simulink model "STLA_6_30"  (R2025a)
settings: Solver=ode3  StartTime=0.0  StopTime=2474  FixedStep=0.01  RelTol=1e-3
model workspace (MAT data in the model file):
  qw = 0.5
libraries: simulink x5, svdutilitieslib x2, instrumentlib x2, autolibshared x1, pid_lib x1
settings Model: Creator=王刚  LastModifiedBy=王刚
settings SolverCC: AlgebraicLoopSolver=TrustRegion
settings RTWCC: DLArmComputeVersion=19.05

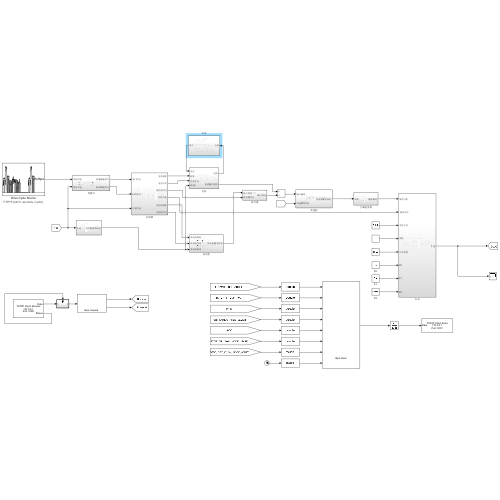
[thumbnail: Simulink's stored preview of the top-level diagram]
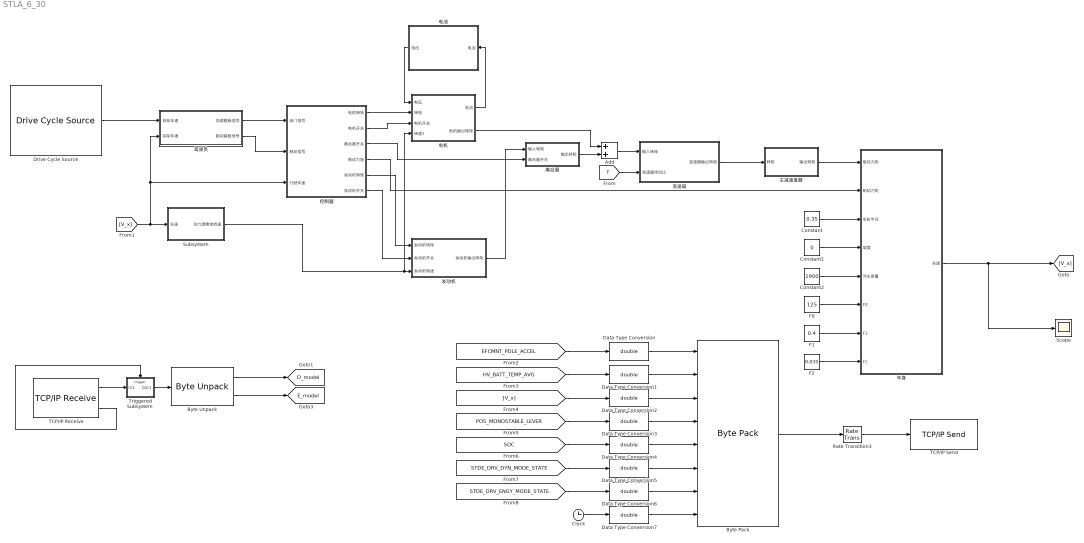
== system STLA_6_30 ==
  Add : Sum
  Byte Pack : svdutilitieslib/Byte Pack  maskPackedDataType=uint8  datatypes={'double', 'double', 'double', 'double', 'double', 'double', 'double', 'double'}  byteAlign=1  blockPlatform=tic2000
  Byte Unpack : svdutilitieslib/Byte Unpack  dimensions={[1] [1]}  datatypes={'double', 'double'}  byteAlign=1  blockPlatform=tic2000
  Clock : Clock
  Constant : Constant  Value=0.35
  Constant1 : Constant  Value=0
  Constant2 : Constant  Value=1900
  Data Type Conversion{,1..7} (8 alike) : DataTypeConversion  OutDataTypeStr=double  SaturateOnIntegerOverflow=off  RndMeth=Floor
  Drive Cycle Source : autolibshared/Drive Cycle Source  cycleVar=FTP75  fileVar=cycleFTP75.mat  tfinal="2474  seconds, Cyclic"  cycleRepeat=on  outAccPort=off  outGearPort=off  gearList=No gear data  t_wot1=5  xdot_woto=0  xdot_wot1=30  t_wot2=20  xdot_wot2=0  t_wotend=30  srcUnit=m/s  outUnit=km/h  srcAccUnit=m/s/s  outAccUnit=m/s^2  dt=0  aMode=1  faultOption=off  velBnd=2  velBndUnit=mph  inUnit=m/s  timeBnd=1  failOption=off  stopSim=off  maxFaultCnt=10  maxFaultTime=2  maxTotFaultTime=15  traceOption=off  dtTrace=1  traceWindow=10  lastDCname=FTP75  lastOutUnit=mph  lastDT=0  lastTB=1  lastSB=2  forceCalcBound=off
  F0 : Constant  Value=125
  F1 : Constant  Value=0.4
  F2 : Constant  Value=0.035
  Rate Transition3 : RateTransition  OutPortSampleTime=0.1
  Scope : Scope
      settings: ActiveDisplayYMinimum=-11.4831  ActiveDisplayYMaximum=103.3483  DataLoggingVariableName=ScopeData5  DataLoggingSaveFormat=Array
  Subsystem : Subsystem
  TCP/IP Receive : instrumentlib/TCP//IP Receive  Host=127.0.0.1  Port=5000  DataSize=16  DataType=uint8  ASCIIFormatting=%f  Terminator=LF  CustomTerminator=10  ByteOrder=big-endian  EnableBlockingMode=off  Timeout=0.01  SampleTime=0.01  SimulateUsing=Interpreted execution
  TCP/IP Send : instrumentlib/TCP//IP Send  Host=127.0.0.1  Port=5001  ByteOrder=big-endian  EnableBlockingMode=off  Timeout=10  TransferDelay=on  SimulateUsing=Interpreted execution
  Triggered Subsystem : Subsystem  TreatAsAtomicUnit=on
  主减速度器 : Subsystem
  发动机 : Subsystem
  变速箱 : Subsystem
  控制器 : Subsystem
  电机 : Subsystem
  电池 : Subsystem
  离合器 : Subsystem
  车身 : Subsystem
  驾驶员 : Subsystem
  tag scope: D_model=global, E_model=global
  wires:
  驾驶员/1(加速踏板信号) -> 控制器/1(油门信号)
  驾驶员/2(制动踏板信号) -> 控制器/2(制动信号)
  Constant/1 -> 车身/3(车轮半径)
  Constant1/1 -> 车身/4(坡度)
  Constant2/1 -> 车身/5(汽车质量)
  F0/1 -> 车身/6(F0)
  F1/1 -> 车身/7(F1)
  F2/1 -> 车身/8(F2)
  变速箱/1(变速器输出转矩) -> 主减速度器/1(转矩)
  主减速度器/1(输出转矩) -> 车身/1("驱动力矩 ")
  控制器/5(发动机转矩) -> 发动机/1(发动机转矩)
  控制器/6(发动机开关) -> 发动机/2(发动机开关)
  控制器/1(电机转矩) -> 电机/2(转矩)
  控制器/2(电机开关) -> 电机/3(电机开关)
  控制器/3(离合器开关) -> 离合器/2(离合器开关)
  控制器/4(制动力矩) -> 车身/2(" 制动力矩")
  电池/1(电压) -> 电机/1(电压)
  离合器/1(输出转矩) -> Add/2
  Add/1 -> 变速箱/1(输入转矩)
  [T] -> 变速箱/2(变速器传动比)
  车身/1(车速) -> [V_x], Scope/1
  [V_x] -> 驾驶员/2(实际车速), 控制器/3(行驶车速), Subsystem/1(车速)
  电机/1(电流) -> 电池/1(电流)
  电机/2(电机输出转矩) -> Add/1
  发动机/1(发动机输出转矩) -> 离合器/1(输入转矩)
  Subsystem/1(动力源需求转速) -> 电机/4(转速1), 发动机/3(发动机转速)
  Drive Cycle Source/1 -> 驾驶员/1(目标车速)
  Triggered Subsystem/1(Out1) -> Byte Unpack/1
  Byte Unpack/1 -> [D_model]
  Byte Unpack/2 -> [E_model]
  TCP/IP Receive/1 -> Triggered Subsystem/1(In1)
  TCP/IP Receive/2 -> Triggered Subsystem/Trigger
  [EFCMNT_PDLE_ACCEL] -> Data Type Conversion/1
  [STDE_DRV_ENGY_MODE_STATE] -> Data Type Conversion6/1
  [STDE_DRV_DYN_MODE_STATE] -> Data Type Conversion5/1
  [SOC] -> Data Type Conversion4/1
  [V_x] -> Data Type Conversion2/1
  [POS_MONOSTABLE_LEVER] -> Data Type Conversion3/1
  [HV_BATT_TEMP_AVG] -> Data Type Conversion1/1
  Byte Pack/1 -> Rate Transition3/1
  Rate Transition3/1 -> TCP/IP Send/1
  Clock/1 -> Data Type Conversion7/1
  Data Type Conversion/1 -> Byte Pack/1
  Data Type Conversion1/1 -> Byte Pack/2
  Data Type Conversion2/1 -> Byte Pack/3
  Data Type Conversion3/1 -> Byte Pack/4
  Data Type Conversion4/1 -> Byte Pack/5
  Data Type Conversion5/1 -> Byte Pack/6
  Data Type Conversion6/1 -> Byte Pack/7
  Data Type Conversion7/1 -> Byte Pack/8

== system STLA_6_30/Subsystem ==
  车速 : Inport
  " " : Constant  Value=0.377
  Product : Product  Inputs=***//
  主减速器传动比 : Constant  Value=4.88
  车轮半径 : Constant  Value=0.25
  动力源需求转速 : Outport
  tag scope: rmp=global
  wires:
  Product/1 -> [rmp], 动力源需求转速/1
  车速/1 -> Product/1
  " "/1 -> Product/5
  主减速器传动比/1 -> Product/2
  车轮半径/1 -> Product/4
  [T] -> Product/3

== system STLA_6_30/Triggered Subsystem ==
  In1 : Inport
  Trigger : TriggerPort  VariantControl=(inherit)
  Out1 : Outport
  wires:
  In1/1 -> Out1/1

== system STLA_6_30/主减速度器 ==
  转矩 : Inport
  Product : Product
  主减速器传动比 : Constant  Value=4.88
  传动效率 : Gain  Gain=0.9
  输出转矩 : Outport
  wires:
  转矩/1 -> Product/1
  主减速器传动比/1 -> Product/2
  Product/1 -> 传动效率/1
  传动效率/1 -> 输出转矩/1

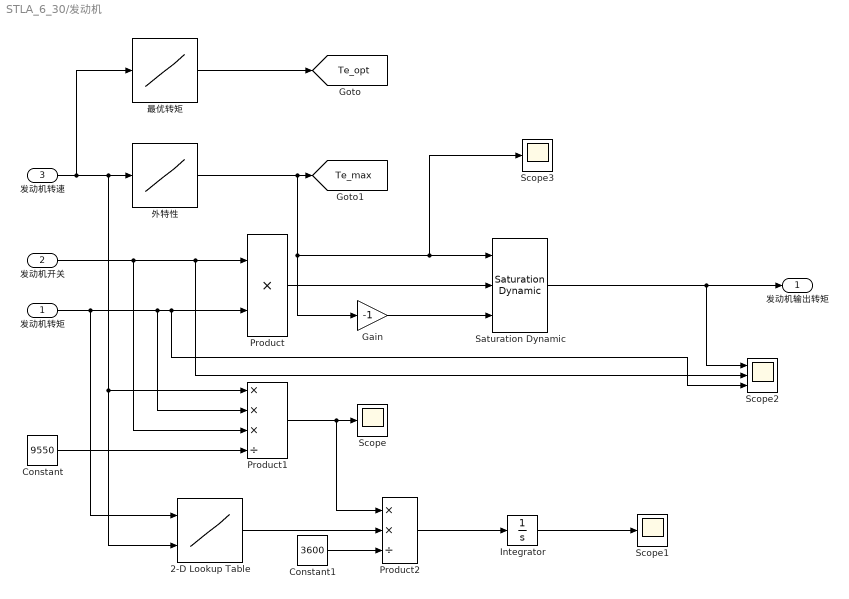
== system STLA_6_30/发动机 ==
  发动机转矩 : Inport
  发动机开关 : Inport  Port=2
  发动机转速 : Inport  Port=3
  2-D Lookup Table : Lookup_n-D  BreakpointsForDimension1=[1000,1500,2000,2500,3000,3500,4000,4500,5000,5500,6000]  BreakpointsForDimension2=[0,25,50,75,100,125,150,175,200,225,250]  Table=|  InternalRulePriority=Speed  RndMeth=Simplest
      | [
      |   800, 600, 500, 450, 420, 400, 400, 420, 450, 500, 600;   % 0 Nm
      |   600, 450, 380, 340, 320, 310, 310, 320, 340, 380, 450;   % 25 Nm
      |   500, 360, 300, 270, 260, 255, 255, 260, 280, 320, 400;   % 50 Nm
      |   480, 320, 265, 240, 230, 225, 225, 230, 250, 290, 370;   % 75 Nm
      |   490, 300, 245, 220, 215, 210, 210, 215, 235, 275, 360;   % 100 Nm
      |   520, 290, 235, 215, 210, 205, 205, 210, 230, 270, 360;   % 125 Nm
      |   580, 300, 240, 220, 215, 210, 210, 215, 240, 280, 380;   % 150 Nm
      |   680, 330, 260, 240, 230, 225, 225, 235, 260, 310, 420;   % 175 Nm
      |   800, 380, 290, 265, 255, 250, 250, 260, 290, 350, 480;   % 200 Nm
      |   NaN, 450, 330, 300, 290, 280, 280, 290, 330, 400, 550;   % 225 Nm（1000rpm 不可达，填 NaN）
      |   NaN, NaN, 380, 350, 340, 330, 330, 340, 390, 470, 650;   % 250 Nm（低转速不可达，填 NaN）
      | ]
      settings: InputPortMap=u0,u1
  Constant : Constant  Value=9550
  Constant1 : Constant  Value=3600
  Gain : Gain  Gain=-1
  Integrator : Integrator
  Product : Product
  Product1 : Product  Inputs=***/
  Product2 : Product  Inputs=**/
  Saturation Dynamic : simulink/Discontinuities/Saturation Dynamic  OutMin=[]  OutMax=[]  OutDataTypeStr=Inherit: Same as second input  OutDataType=fixdt(1, 16)  OutScaling=2^-10  DoSatur=off
  Scope : Scope
      settings: ActiveDisplayYMinimum=-1  ActiveDisplayYMaximum=1  DataLoggingVariableName=ScopeData4  DataLoggingSaveFormat=Array
  Scope1 : Scope
      settings: ActiveDisplayYMinimum=-1  ActiveDisplayYMaximum=1  DataLoggingVariableName=ScopeData10  DataLoggingSaveFormat=Array
  Scope2 : Scope  NumInputPorts=3
      settings: ActiveDisplayYMinimum=-45  ActiveDisplayYMaximum=405  DataLoggingVariableName=ScopeData20  DataLoggingSaveFormat=Array
  Scope3 : Scope
      settings: ActiveDisplayYMinimum=-1  ActiveDisplayYMaximum=1  DataLoggingVariableName=ScopeData21  DataLoggingSaveFormat=Array
  外特性 : Lookup_n-D  NumberOfTableDimensions=1  BreakpointsForDimension1="[1000  1500  2000  2500  3000  3500  4000  4500  5000  5500  6000]"  Table="[125   187   250   250   250   250   250   250   210   191   175]"  InternalRulePriority=Speed  RndMeth=Simplest
  最优转矩 : Lookup_n-D  NumberOfTableDimensions=1  BreakpointsForDimension1="[1000  1500  2000  2500  3000  3500  4000  4500  5000  5500  6000]"  Table="[80    115   150   150   150   150   150   150   140   130   120]"  InternalRulePriority=Speed  RndMeth=Simplest
  发动机输出转矩 : Outport
  tag scope: Te_max=global, Te_opt=global
  wires:
  Constant/1 -> Product1/4
  Product1/1 -> Product2/1, Scope/1
  发动机开关/1 -> Scope2/2, Product/1, Product1/3
  发动机转速/1 -> 最优转矩/1, Product1/1, 2-D Lookup Table/2, 外特性/1
  最优转矩/1 -> [Te_opt]
  外特性/1 -> Gain/1, Scope3/1, Saturation Dynamic/1, [Te_max]
  发动机转矩/1 -> 2-D Lookup Table/1, Product1/2, Scope2/3, Product/2
  Saturation Dynamic/1 -> Scope2/1, 发动机输出转矩/1
  Product/1 -> Saturation Dynamic/2
  Gain/1 -> Saturation Dynamic/3
  2-D Lookup Table/1 -> Product2/2
  Constant1/1 -> Product2/3
  Product2/1 -> Integrator/1
  Integrator/1 -> Scope1/1

== system STLA_6_30/变速箱 ==
  输入转矩 : Inport
  变速器传动比 : Inport  Port=2
  Product : Product
  变速器输出转矩 : Outport
  wires:
  输入转矩/1 -> Product/1
  变速器传动比/1 -> Product/2
  Product/1 -> 变速器输出转矩/1

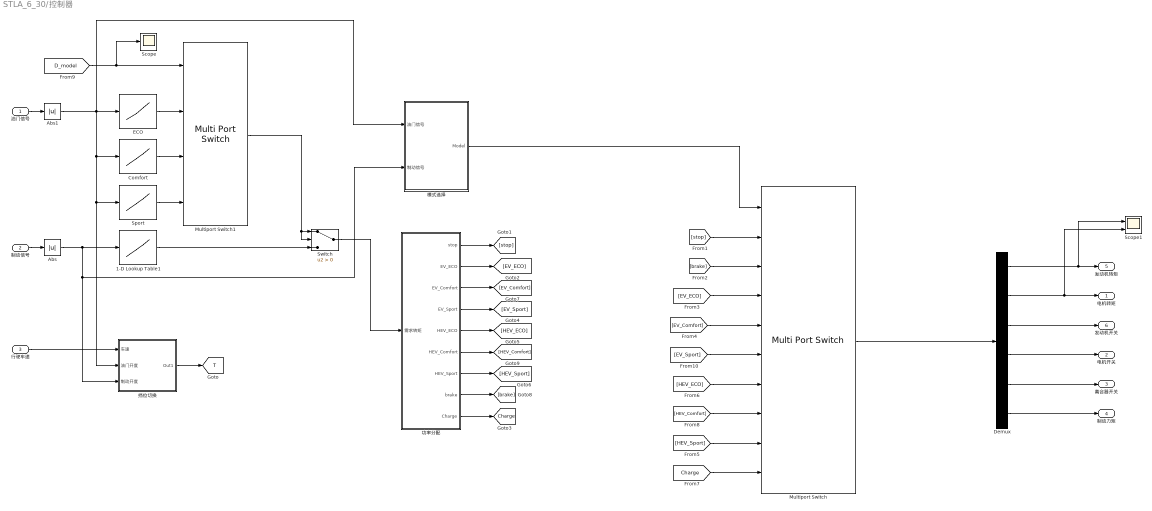
== system STLA_6_30/控制器 ==
  油门信号 : Inport
  制动信号 : Inport  Port=2
  行驶车速 : Inport  Port=3
  1-D Lookup Table1 : Lookup_n-D  NumberOfTableDimensions=1  BreakpointsForDimension1=[0 0.1 0.3 0.5 0.7 0.9 1.0]  Table=[0 30 90 150 210 270 300]  InternalRulePriority=Speed  RndMeth=Simplest
  Abs : Abs  ZeroCross=off  SaturateOnIntegerOverflow=off
  Abs1 : Abs  ZeroCross=off  SaturateOnIntegerOverflow=off
  Comfort : Lookup_n-D  NumberOfTableDimensions=1  BreakpointsForDimension1=[0 0.1 0.2 0.3 0.4 0.5 0.6 0.7 0.8 0.9 1.0]  Table=[0 36 72 108 144 180 216 252 288 324 360]  InternalRulePriority=Speed  RndMeth=Simplest
  Demux : Demux  Outputs=6
  ECO : Lookup_n-D  NumberOfTableDimensions=1  BreakpointsForDimension1=[0 0.1 0.2 0.3 0.4 0.5 0.6 0.7 0.8 0.9 1.0]  Table=[0 15 30 50 75 105 140 180 225 270 310]  InternalRulePriority=Speed  RndMeth=Simplest
  Multiport Switch : MultiPortSwitch  Inputs=9  SaturateOnIntegerOverflow=off  InputSameDT=off
  Multiport Switch1 : MultiPortSwitch  DataPortOrder=Zero-based contiguous  DiagnosticForDefault=None  zeroidx=on  SaturateOnIntegerOverflow=off  InputSameDT=off
  Scope : Scope
      settings: ActiveDisplayYMinimum=-1  ActiveDisplayYMaximum=1  DataLoggingVariableName=ScopeData9  DataLoggingSaveFormat=Array
  Scope1 : Scope  NumInputPorts=2
      settings: ActiveDisplayYMinimum=-326.2466  ActiveDisplayYMaximum=436.2496  DataLoggingVariableName=ScopeData19  DataLoggingSaveFormat=Array
  Sport : Lookup_n-D  NumberOfTableDimensions=1  BreakpointsForDimension1=[0 0.1 0.2 0.3 0.4 0.5 0.6 0.7 0.8 0.9 1.0]  Table=[0 75 150 220 280 320 345 355 360 360 360]  InternalRulePriority=Speed  RndMeth=Simplest
  Switch : Switch  Criteria=u2 > Threshold  ZeroCross=off  SaturateOnIntegerOverflow=off  InputSameDT=off
  功率分配 : Subsystem
  挡位切换 : Subsystem
  模式选择 : Subsystem
  电机转矩 : Outport
  电机开关 : Outport  Port=2
  离合器开关 : Outport  Port=3
  制动力矩 : Outport  Port=4
  发动机转矩 : Outport  Port=5
  发动机开关 : Outport  Port=6
  tag scope: Charge=global, T=global
  wires:
  油门信号/1 -> Abs1/1
  制动信号/1 -> Abs/1
  Abs/1 -> 模式选择/2(制动信号), 挡位切换/3(制动开度), 1-D Lookup Table1/1
  1-D Lookup Table1/1 -> Switch/3
  ECO/1 -> Multiport Switch1/2
  Switch/1 -> 功率分配/1(需求转矩)
  行驶车速/1 -> 挡位切换/1(车速)
  功率分配/1(stop) -> [stop]
  功率分配/2(EV_ECO) -> [EV_ECO]
  [stop] -> Multiport Switch/2
  [brake] -> Multiport Switch/3
  [EV_Comfort] -> Multiport Switch/5
  [EV_Sport] -> Multiport Switch/6
  [HEV_ECO] -> Multiport Switch/7
  [EV_ECO] -> Multiport Switch/4
  Multiport Switch/1 -> Demux/1
  Demux/1 -> Scope1/1, 发动机转矩/1
  Demux/2 -> Scope1/2, 电机转矩/1
  Demux/3 -> 发动机开关/1
  Demux/4 -> 电机开关/1
  Demux/5 -> 离合器开关/1
  Demux/6 -> 制动力矩/1
  模式选择/1(Model) -> Multiport Switch/1
  功率分配/3(EV_Comfort) -> [EV_Comfort]
  功率分配/4(EV_Sport) -> [EV_Sport]
  功率分配/5(HEV_ECO) -> [HEV_ECO]
  功率分配/7(HEV_Sport) -> [HEV_Sport]
  功率分配/6(HEV_Comfort) -> [HEV_Comfort]
  功率分配/8(brake) -> [brake]
  [HEV_Comfort] -> Multiport Switch/8
  [HEV_Sport] -> Multiport Switch/9
  挡位切换/1(Out1) -> [T]
  Comfort/1 -> Multiport Switch1/3
  Sport/1 -> Multiport Switch1/4
  [D_model] -> Scope/1, Multiport Switch1/1
  Multiport Switch1/1 -> Switch/2, Switch/1
  功率分配/9(Charge) -> [Charge]
  [Charge] -> Multiport Switch/10
  Abs1/1 -> 模式选择/1(油门信号), 挡位切换/2(油门开度), Sport/1, Comfort/1, ECO/1

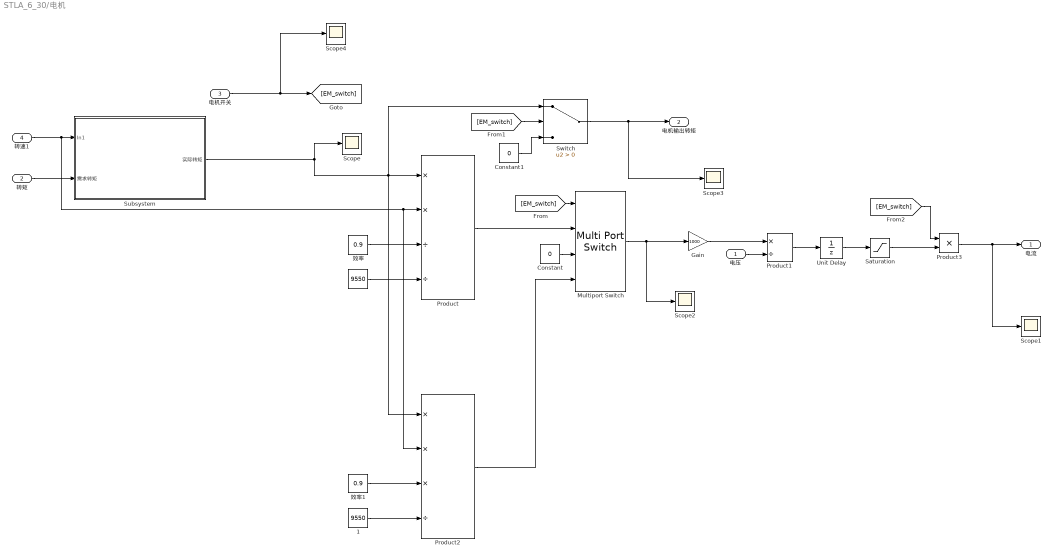
== system STLA_6_30/电机 ==
  电压 : Inport
  转矩 : Inport  Port=2
  电机开关 : Inport  Port=3
  转速1 : Inport  Port=4
  " " : Constant  Value=9550
  " 1" : Constant  Value=9550
  Constant : Constant  Value=0
  Constant1 : Constant  Value=0
  Gain : Gain  Gain=1000
  Multiport Switch : MultiPortSwitch  DataPortOrder=Specify indices  DataPortIndices={1,0,-1}  SaturateOnIntegerOverflow=off  InputSameDT=off
  Product : Product  Inputs=**//
  Product1 : Product  Inputs=*/
  Product2 : Product  Inputs=***/
  Product3 : Product
  Saturation : Saturate  UpperLimit=250  LowerLimit=-250  ZeroCross=off
  Scope{,1..4} (5 alike) : Scope
      Scope settings: ActiveDisplayYMinimum=-13.75  ActiveDisplayYMaximum=123.75  DataLoggingVariableName=ScopeData11  DataLoggingSaveFormat=Array
      Scope1 settings: ActiveDisplayYMinimum=-249.3565  ActiveDisplayYMaximum=249.5466  DataLoggingVariableName=ScopeData7  DataLoggingSaveFormat=Array
      Scope2 settings: ActiveDisplayYMinimum=-4.9486  ActiveDisplayYMaximum=44.5371  DataLoggingVariableName=ScopeData12  DataLoggingSaveFormat=Array
      Scope3 settings: ActiveDisplayYMinimum=-13.75  ActiveDisplayYMaximum=123.75  DataLoggingVariableName=ScopeData14  DataLoggingSaveFormat=Array
      Scope4 settings: ActiveDisplayYMinimum=-1.25  ActiveDisplayYMaximum=1.25  DataLoggingVariableName=ScopeData15  DataLoggingSaveFormat=Array
  Subsystem : Subsystem
  Switch : Switch  Criteria=u2 > Threshold  ZeroCross=off  SaturateOnIntegerOverflow=off  InputSameDT=off
  Unit Delay : UnitDelay  SampleTime=-1  HasFrameUpgradeWarning=on
  效率 : Constant  Value=0.9
  效率1 : Constant  Value=0.9
  电流 : Outport
  电机输出转矩 : Outport  Port=2
  wires:
  效率/1 -> Product/3
  " "/1 -> Product/4
  Gain/1 -> Product1/1
  电压/1 -> Product1/2
  Product1/1 -> Unit Delay/1
  Unit Delay/1 -> Saturation/1
  转速1/1 -> Product2/2, Product/2, Subsystem/1(In1)
  效率1/1 -> Product2/3
  " 1"/1 -> Product2/4
  Constant/1 -> Multiport Switch/3
  Product/1 -> Multiport Switch/2
  Product2/1 -> Multiport Switch/4
  电机开关/1 -> Scope4/1, [EM_switch]
  [EM_switch] -> Multiport Switch/1
  [EM_switch] -> Switch/2
  Constant1/1 -> Switch/3
  Switch/1 -> Scope3/1, 电机输出转矩/1
  Multiport Switch/1 -> Scope2/1, Gain/1
  Subsystem/1(实际转矩) -> Scope/1, Product/1, Switch/1, Product2/1
  转矩/1 -> Subsystem/2(需求转矩)
  Product3/1 -> Scope1/1, 电流/1
  Saturation/1 -> Product3/2
  [EM_switch] -> Product3/1

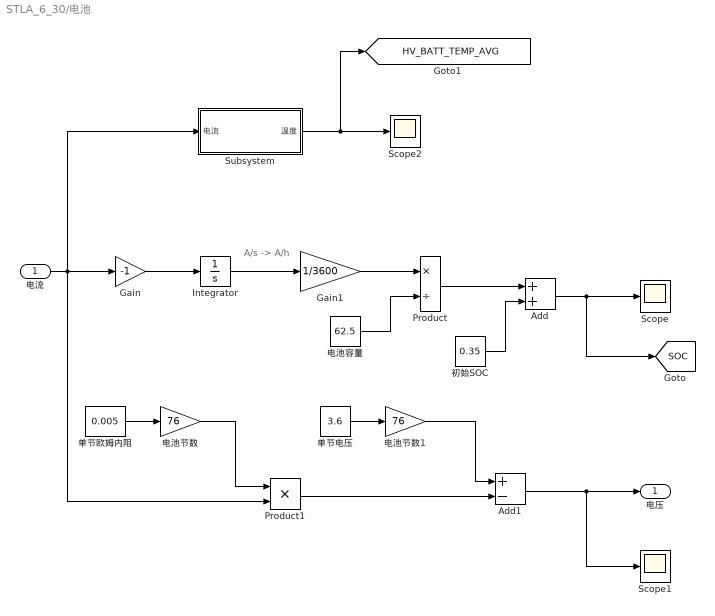
== system STLA_6_30/电池 ==
  note: A/s -> A/h
  电流 : Inport
  Add : Sum
  Add1 : Sum  Inputs=+-
  Gain : Gain  Gain=-1
  Gain1 : Gain  Gain=1/3600
  Integrator : Integrator
  Product : Product  Inputs=*/
  Product1 : Product
  Scope : Scope
      settings: ActiveDisplayYMinimum=0.18682  ActiveDisplayYMaximum=0.3185  DataLoggingVariableName=ScopeData2  DataLoggingSaveFormat=Array
  Scope1 : Scope
      settings: ActiveDisplayYMinimum=188.2402  ActiveDisplayYMaximum=283.0844  DataLoggingVariableName=ScopeData8  DataLoggingSaveFormat=Array
  Scope2 : Scope
      settings: ActiveDisplayYMinimum=19.7986  ActiveDisplayYMaximum=59.9395  DataLoggingSaveFormat=Array
  Subsystem : Subsystem
  初始SOC : Constant  Value=0.35
  单节欧姆内阻 : Constant  Value=0.005
  单节电压 : Constant  Value=3.6
  电池容量 : Constant  Value=62.5
  电池节数 : Gain  Gain=76
  电池节数1 : Gain  Gain=76
  电压 : Outport
  tag scope: HV_BATT_TEMP_AVG=global, SOC=global
  wires:
  Gain/1 -> Integrator/1
  Integrator/1 -> Gain1/1
  Gain1/1 -> Product/1
  电池容量/1 -> Product/2
  Product/1 -> Add/1
  初始SOC/1 -> Add/2
  Add/1 -> [SOC], Scope/1
  电流/1 -> Subsystem/1(电流), Product1/2, Gain/1
  单节欧姆内阻/1 -> 电池节数/1
  电池节数/1 -> Product1/1
  单节电压/1 -> 电池节数1/1
  电池节数1/1 -> Add1/1
  Product1/1 -> Add1/2
  Add1/1 -> Scope1/1, 电压/1
  Subsystem/1(温度) -> [HV_BATT_TEMP_AVG], Scope2/1

== system STLA_6_30/离合器 ==
  输入转矩 : Inport
  离合器开关 : Inport  Port=2
  Product : Product
  输出转矩 : Outport
  wires:
  输入转矩/1 -> Product/1
  离合器开关/1 -> Product/2
  Product/1 -> 输出转矩/1

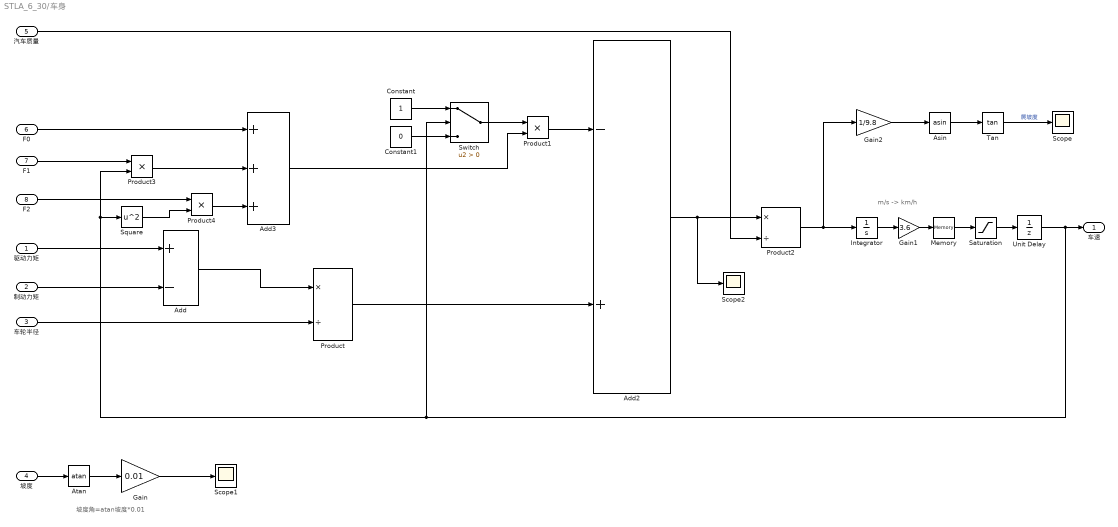
== system STLA_6_30/车身 ==
  note: m/s -> km/h
  note: 坡度角=atan坡度*0.01
  "驱动力矩 " : Inport
  " 制动力矩" : Inport  Port=2
  车轮半径 : Inport  Port=3
  坡度 : Inport  Port=4
  汽车质量 : Inport  Port=5
  F0 : Inport  Port=6
  F1 : Inport  Port=7
  F2 : Inport  Port=8
  Add : Sum  Inputs=+-
  Add2 : Sum  Inputs=-+
  Add3 : Sum  Inputs=+++
  Asin : Trigonometry  Operator=asin
  Atan : Trigonometry  Operator=atan
  Constant : Constant
  Constant1 : Constant  Value=0
  Gain : Gain  Gain=0.01
  Gain1 : Gain  Gain=3.6
  Gain2 : Gain  Gain=1/9.8
  Integrator : Integrator  ZeroCross=off
  Memory : Memory
  Product : Product  Inputs=*/
  Product1 : Product
  Product2 : Product  Inputs=*/
  Product3 : Product
  Product4 : Product
  Saturation : Saturate  UpperLimit=100000  LowerLimit=0  ZeroCross=off
  Scope : Scope
      settings: DataLoggingVariableName=ScopeData3  DataLoggingSaveFormat=Array
  Scope1 : Scope
      settings: ActiveDisplayYMinimum=-1  ActiveDisplayYMaximum=1  DataLoggingVariableName=ScopeData13  DataLoggingSaveFormat=Array
  Scope2 : Scope
      settings: ActiveDisplayYMinimum=-2906.8903  ActiveDisplayYMaximum=13947.9387  DataLoggingVariableName=ScopeData18  DataLoggingSaveFormat=Array
  Square : Math  Operator=square
  Switch : Switch  Criteria=u2 > Threshold  SaturateOnIntegerOverflow=off  InputSameDT=off
  Tan : Trigonometry  Operator=tan
  Unit Delay : UnitDelay  SampleTime=-1  HasFrameUpgradeWarning=on
  车速 : Outport
  wires:
  "驱动力矩 "/1 -> Add/1
  " 制动力矩"/1 -> Add/2
  Add/1 -> Product/1
  车轮半径/1 -> Product/2
  坡度/1 -> Atan/1
  Atan/1 -> Gain/1
  汽车质量/1 -> Product2/2
  Switch/1 -> Product1/1
  Constant/1 -> Switch/1
  Constant1/1 -> Switch/3
  Product1/1 -> Add2/1
  Product/1 -> Add2/2
  Add2/1 -> Scope2/1, Product2/1
  Product2/1 -> Gain2/1, Integrator/1
  Gain1/1 -> Memory/1
  Saturation/1 -> Unit Delay/1
  Add3/1 -> Product1/2
  Gain2/1 -> Asin/1
  Asin/1 -> Tan/1
  Tan/1 -> Scope/1  "爬坡度"
  Gain/1 -> Scope1/1
  F0/1 -> Add3/1
  F1/1 -> Product3/1
  F2/1 -> Product4/1
  Integrator/1 -> Gain1/1
  Square/1 -> Product4/2
  Product3/1 -> Add3/2
  Product4/1 -> Add3/3
  Unit Delay/1 -> 车速/1, Square/1, Product3/2, Switch/2
  Memory/1 -> Saturation/1

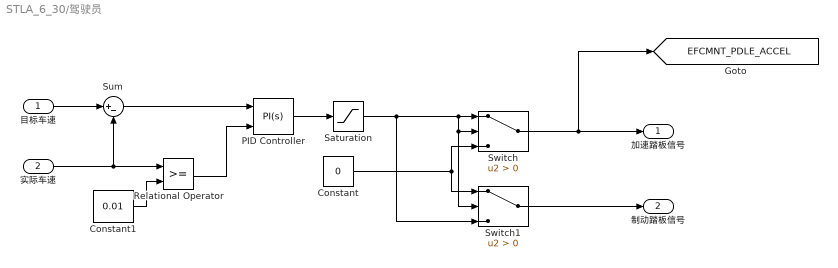
== system STLA_6_30/驾驶员 ==
  目标车速 : Inport
  实际车速 : Inport  Port=2
  Constant : Constant  Value=0
  Constant1 : Constant  Value=0.01
  PID Controller : pid_lib/PID Controller  Controller=PI  Form=Parallel  TimeDomain=Continuous-time  UseExternalTs=off  SampleTime=-1  IntegratorMethod=Forward Euler  ControllerParametersSource=internal  P=0.5  I=0.06  D=0  N=100  UseFilter=on  TunerSelectOption=Transfer Function Based (PID Tuner App)  InitialConditionSource=internal  InitialConditionForIntegrator=0  InitialConditionForFilter=0  DifferentiatorICPrevScaledInput=0  ExternalReset=falling  TrackingMode=off  Kt=1  LimitOutput=off  SatLimitsSource=internal  UpperSaturationLimit=inf  LowerSaturationLimit=-inf  LinearizeAsGain=on  AntiWindupMode=none  Kb=1  POutMin=[]  POutMax=[]  IOutMin=[]  IOutMax=[]  DOutMin=[]  DOutMax=[]  NOutMin=[]  NOutMax=[]  SumOutMin=[]  SumOutMax=[]  SaturationOutMin=[]  SaturationOutMax=[]  PParamMin=[]  PParamMax=[]  IParamMin=[]  IParamMax=[]  DParamMin=[]  DParamMax=[]  NParamMin=[]  NParamMax=[]  KbParamMin=[]  KbParamMax=[]  KtParamMin=[]  KtParamMax=[]  KbOutMin=[]  KbOutMax=[]  KtOutMin=[]  KtOutMax=[]  IntegratorOutMin=[]  IntegratorOutMax=[]  FilterOutMin=[]  FilterOutMax=[]  SumI1OutMin=[]  SumI1OutMax=[]  SumI2OutMin=[]  SumI2OutMax=[]  SumI3OutMin=[]  SumI3OutMax=[]  SumI4OutMin=[]  SumI4OutMax=[]  SumDOutMin=[]  SumDOutMax=[]  DifferentiatorOutMin=[]  DifferentiatorOutMax=[]  FilterDiffOutCoefMin=[]  FilterDiffOutCoefMax=[]  ReciprocalOutMin=[]  ReciprocalOutMax=[]  SumDenOutMin=[]  SumDenOutMax=[]  SumNumOutMin=[]  SumNumOutMax=[]  DivideOutMin=[]  DivideOutMax=[]  UdiffTsProdOutMin=[]  UdiffTsProdOutMax=[]  NTsProdOutMin=[]  NTsProdOutMax=[]  UintegralTsProdOutMin=[]  UintegralTsProdOutMax=[]  UngainTsProdOutMin=[]  UngainTsProdOutMax=[]  IntegratorContinuousStateAttributes=''  IntegratorStateMustResolveToSignalObject=off  IntegratorRTWStateStorageClass=Auto  FilterContinuousStateAttributes=''  FilterStateMustResolveToSignalObject=off  FilterRTWStateStorageClass=Auto  ParallelPVariant=InternalParameters  IdealPVariant=Disabled  IVariant=InternalParameters  DVariant=Disabled  IntegratorVariant=Continuous  SatVariant=Disabled  AWVariant=Passthrough  PCopyVariant=Disabled  TRVariant=Disabled  FdbkBlocksVariant=Forward  IdealPFdbkVariant=Disabled  SatFdbkVariant=Disabled  DerivativeFilterVariant=Disabled  NVariant=Disabled  NCopyVariant=Disabled_SignalSpec  FilterICVariant=Disabled  IntegratorICVariant=InternalICs  ExternalResetVariant=ExternalReset  TRSumVariant=Passthrough  SumFdbkVariant=Disabled  SumVariant=Sum_PI  TsampFilterVariant=InternalTs  TsampNgainVariant=Passthrough  TsampIntegralVariant=Disabled_SignalSpec  ExternalSaturationOutDataTypeStr=Inherit: Same as second input
  Relational Operator : RelationalOperator  OutDataTypeStr=boolean  RndMeth=Simplest  InputSameDT=off
  Saturation : Saturate  UpperLimit=1  LowerLimit=-1
  Sum : Sum  Inputs=|+-
  Switch : Switch  Criteria=u2 > Threshold  ZeroCross=off  SaturateOnIntegerOverflow=off  InputSameDT=off
  Switch1 : Switch  Criteria=u2 > Threshold  ZeroCross=off  SaturateOnIntegerOverflow=off  InputSameDT=off
  加速踏板信号 : Outport
  制动踏板信号 : Outport  Port=2
  tag scope: EFCMNT_PDLE_ACCEL=global
  wires:
  目标车速/1 -> Sum/1
  实际车速/1 -> Sum/2, Relational Operator/1
  Sum/1 -> PID Controller/1
  PID Controller/1 -> Saturation/1
  Saturation/1 -> Switch1/3, Switch1/2, Switch/2, Switch/1
  Switch/1 -> [EFCMNT_PDLE_ACCEL], 加速踏板信号/1
  Switch1/1 -> 制动踏板信号/1
  Constant/1 -> Switch/3, Switch1/1
  Relational Operator/1 -> PID Controller/2
  Constant1/1 -> Relational Operator/2

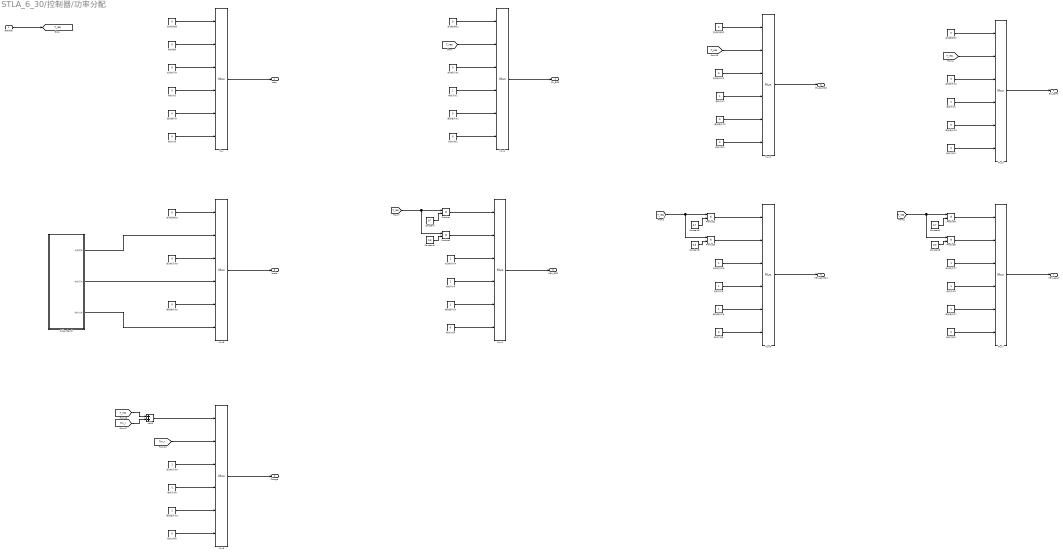
== system STLA_6_30/控制器/功率分配 ==
  需求转矩 : Inport
  Add5 : Sum
  Constant : Constant  Value=0.7
  Constant1 : Constant  Value=0.3
  Constant2 : Constant  Value=0.7
  Constant3 : Constant  Value=0.3
  Constant4 : Constant  Value=0.7
  Constant5 : Constant  Value=0.3
  Mux{,1..8} (9 alike) : Mux  Inputs=6
  Product{,1..5} (6 alike) : Product
  Subsystem3 : Subsystem
  制动力矩{,1..6,9} (8 alike) : Constant  Value=0
  发动机开关{,1..3,5} (5 alike) : Constant  Value=0
  发动机开关{4,6..7,9} (4 alike) : Constant
  发动机转矩{,1..3,5} (5 alike) : Constant  Value=0
  电机开关 : Constant  Value=0
  电机开关{1..6} (6 alike) : Constant
  电机开关9 : Constant  Value=-1
  电机转矩 : Constant  Value=0
  离合器开关{,1..3,5} (5 alike) : Constant  Value=0
  离合器开关{4,6..7,9} (4 alike) : Constant
  stop : Outport
  EV_ECO : Outport  Port=2
  EV_Comfort : Outport  Port=3
  EV_Sport : Outport  Port=4
  HEV_ECO : Outport  Port=5
  HEV_Comfort : Outport  Port=6
  HEV_Sport : Outport  Port=7
  brake : Outport  Port=8
  Charge : Outport  Port=9
  tag scope: T_req=global
  wires:
  需求转矩/1 -> [T_req]
  发动机转矩/1 -> Mux/1
  发动机开关/1 -> Mux/3
  电机转矩/1 -> Mux/2
  电机开关/1 -> Mux/4
  制动力矩/1 -> Mux/6
  离合器开关/1 -> Mux/5
  Mux/1 -> stop/1
  离合器开关1/1 -> Mux1/5
  Mux1/1 -> EV_ECO/1
  制动力矩1/1 -> Mux1/6
  发动机转矩1/1 -> Mux1/1
  发动机开关1/1 -> Mux1/3
  电机开关1/1 -> Mux1/4
  Mux4/1 -> HEV_ECO/1
  制动力矩4/1 -> Mux4/6
  Mux5/1 -> brake/1
  发动机转矩5/1 -> Mux5/1
  离合器开关5/1 -> Mux5/5
  发动机开关5/1 -> Mux5/3
  [T_req] -> Mux1/2
  发动机开关2/1 -> Mux2/3
  离合器开关2/1 -> Mux2/5
  制动力矩2/1 -> Mux2/6
  Mux2/1 -> EV_Comfort/1
  发动机转矩2/1 -> Mux2/1
  电机开关2/1 -> Mux2/4
  Mux3/1 -> EV_Sport/1
  制动力矩3/1 -> Mux3/6
  发动机转矩3/1 -> Mux3/1
  离合器开关3/1 -> Mux3/5
  电机开关3/1 -> Mux3/4
  发动机开关3/1 -> Mux3/3
  Mux6/1 -> HEV_Comfort/1
  Mux7/1 -> HEV_Sport/1
  [T_req] -> Mux2/2
  [T_req] -> Mux3/2
  Subsystem3/1(电机转矩) -> Mux5/2
  Mux8/1 -> Charge/1
  离合器开关9/1 -> Mux8/5
  发动机开关9/1 -> Mux8/3
  电机开关9/1 -> Mux8/4
  [Tm_r] -> Mux8/2
  [Tm_r] -> Add5/2
  [T_req] -> Add5/1
  Add5/1 -> Mux8/1
  制动力矩9/1 -> Mux8/6
  Subsystem3/2(电机开关) -> Mux5/4
  Subsystem3/3("制动力矩 ") -> Mux5/6
  发动机开关4/1 -> Mux4/3
  电机开关4/1 -> Mux4/4
  离合器开关4/1 -> Mux4/5
  离合器开关6/1 -> Mux6/5
  电机开关5/1 -> Mux6/4
  发动机开关6/1 -> Mux6/3
  制动力矩5/1 -> Mux6/6
  制动力矩6/1 -> Mux7/6
  离合器开关7/1 -> Mux7/5
  [T_req] -> Product1/1, Product/1
  Product1/1 -> Mux4/2
  Product/1 -> Mux4/1
  Constant1/1 -> Product1/2
  Constant/1 -> Product/2
  Constant2/1 -> Product2/2
  Constant3/1 -> Product3/2
  Product2/1 -> Mux6/1
  Product3/1 -> Mux6/2
  [T_req] -> Product2/1, Product3/1
  [T_req] -> Product5/1, Product4/1
  Product5/1 -> Mux7/2
  Product4/1 -> Mux7/1
  Constant5/1 -> Product5/2
  Constant4/1 -> Product4/2
  发动机开关7/1 -> Mux7/3
  电机开关6/1 -> Mux7/4

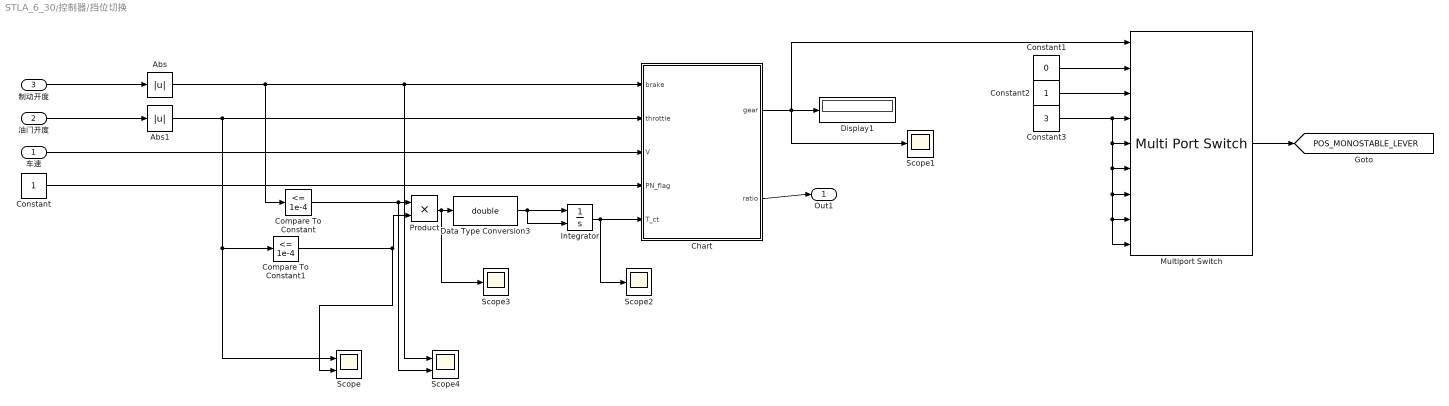
== system STLA_6_30/控制器/挡位切换 ==
  车速 : Inport
  油门开度 : Inport  Port=2
  制动开度 : Inport  Port=3
  Abs : Abs  SaturateOnIntegerOverflow=off
  Abs1 : Abs  SaturateOnIntegerOverflow=off
  Chart : Stateflow chart  TreatAsAtomicUnit=on
  Compare To Constant : simulink/Logic and Bit Operations/Compare To Constant  relop=<=  const=1e-4  OutDataTypeStr=boolean
  Compare To Constant1 : simulink/Logic and Bit Operations/Compare To Constant  relop=<=  const=1e-4  OutDataTypeStr=boolean
  Constant : Constant
  Constant1 : Constant  Value=0
  Constant2 : Constant
  Constant3 : Constant  Value=3
  Data Type Conversion3 : DataTypeConversion  OutDataTypeStr=double  SaturateOnIntegerOverflow=off  RndMeth=Floor
  Display1 : Display
  Integrator : Integrator  ExternalReset=either
  Multiport Switch : MultiPortSwitch  DataPortOrder=Zero-based contiguous  Inputs=8  zeroidx=on  SaturateOnIntegerOverflow=off  InputSameDT=off
  Product : Product
  Scope : Scope  NumInputPorts=2
      settings: ActiveDisplayYMinimum=-0.125  ActiveDisplayYMaximum=1.125  DataLoggingVariableName=ScopeData24  DataLoggingSaveFormat=Array
  Scope1 : Scope
      settings: ActiveDisplayYMinimum=-0.75  ActiveDisplayYMaximum=6.75  DataLoggingVariableName=ScopeData6  DataLoggingSaveFormat=Array
  Scope2 : Scope
      settings: ActiveDisplayYMinimum=-191.0751  ActiveDisplayYMaximum=711.2365  DataLoggingSaveFormat=Array
  Scope3 : Scope
      settings: ActiveDisplayYMinimum=-4.0772  ActiveDisplayYMaximum=6.7431  DataLoggingVariableName=ScopeData22  DataLoggingSaveFormat=Array
  Scope4 : Scope  NumInputPorts=2
      settings: ActiveDisplayYMinimum=-1.25  ActiveDisplayYMaximum=1.25  DataLoggingVariableName=ScopeData25  DataLoggingSaveFormat=Array
  Out1 : Outport
  tag scope: POS_MONOSTABLE_LEVER=global
  wires:
  油门开度/1 -> Abs1/1
  Chart/2(ratio) -> Out1/1
  Chart/1(gear) -> Multiport Switch/1, Scope1/1, Display1/1
  制动开度/1 -> Abs/1
  车速/1 -> Chart/3(V)
  Data Type Conversion3/1 -> Integrator/1, Integrator/2
  Constant/1 -> Chart/4(PN_flag)
  Integrator/1 -> Scope2/1, Chart/5(T_ct)
  Compare To Constant/1 -> Scope4/2, Product/1
  Compare To Constant1/1 -> Scope/2, Product/2
  Product/1 -> Scope3/1, Data Type Conversion3/1
  Multiport Switch/1 -> [POS_MONOSTABLE_LEVER]
  Constant1/1 -> Multiport Switch/2
  Constant3/1 -> Multiport Switch/6, Multiport Switch/7, Multiport Switch/9, Multiport Switch/8, Multiport Switch/5, Multiport Switch/4
  Constant2/1 -> Multiport Switch/3
  Abs/1 -> Scope4/1, Chart/1(brake), Compare To Constant/1
  Abs1/1 -> Chart/2(throttle), Compare To Constant1/1, Scope/1

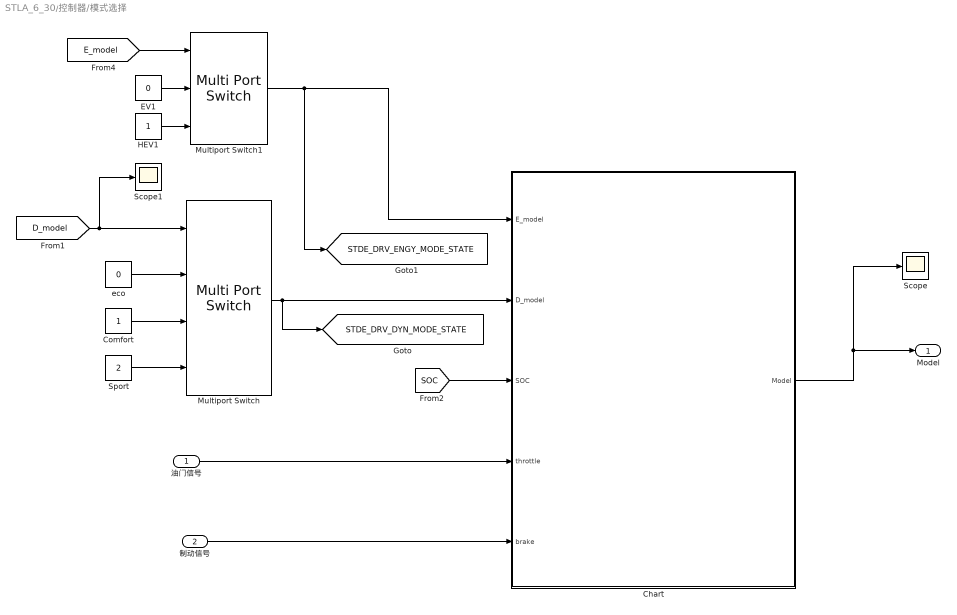
== system STLA_6_30/控制器/模式选择 ==
  油门信号 : Inport
  制动信号 : Inport  Port=2
  Chart : Stateflow chart  TreatAsAtomicUnit=on
      settings: PortSchema="{\"entries\":[{\"content\":{\"sides\":[{\"content\":{\"connectorIds\":[\"In3\",\"In4\",\"In5\",\"In1\",\"In2\"]},\"type\":\"ConnectorPlacement.EquallySpacedRectSide\",\"uuid\":\"a71f6391-e1d2-4931-91ac-1713c8a3738f\"},{\"content\":{\"connectorIds\":[\"Out1\"],\"side\":\"RIGHT\"},\"type\":\"ConnectorPlacement.EquallySpacedRectSide\",\"uuid\":\"fe57e218-1817-4c39-bfc1-b40cd5d4e9a9\"},{\"content\":{\"side\":\"TOP\"},\"type\":\"ConnectorPlacement.EquallySpacedRectSide\",\"uuid\":\"be5ec62b-3236-4b8b-9d89-5acfc240f42d\"}]},\"type\":\"ConnectorPlacement.EquallySpacedConnector\",\"uuid\":\"de164ca6-ce59-445c-bbbb-698006a1e93c\"}],\"packageUris\":[\"http://schema.mathworks.com/mf0/Connector/R2020b\"],\"version\":\"1.0\"}"
  Comfort : Constant
  EV1 : Constant  Value=0
  HEV1 : Constant
  Multiport Switch : MultiPortSwitch  DataPortOrder=Zero-based contiguous  DiagnosticForDefault=None  zeroidx=on  SaturateOnIntegerOverflow=off  InputSameDT=off
  Multiport Switch1 : MultiPortSwitch  DataPortOrder=Zero-based contiguous  Inputs=2  DiagnosticForDefault=None  zeroidx=on  SaturateOnIntegerOverflow=off  InputSameDT=off
  Scope : Scope
      settings: ActiveDisplayYMinimum=-0.34149  ActiveDisplayYMaximum=10.2191  DataLoggingVariableName=ScopeData16  DataLoggingSaveFormat=Array
  Scope1 : Scope
      settings: ActiveDisplayYMinimum=0.9  ActiveDisplayYMaximum=1.1  DataLoggingVariableName=ScopeData23  DataLoggingSaveFormat=Array
  Sport : Constant  Value=2
  eco : Constant  Value=0
  Model : Outport
  tag scope: STDE_DRV_DYN_MODE_STATE=global, STDE_DRV_ENGY_MODE_STATE=global
  wires:
  eco/1 -> Multiport Switch/2
  Comfort/1 -> Multiport Switch/3
  Sport/1 -> Multiport Switch/4
  [D_model] -> Scope1/1, Multiport Switch/1
  Multiport Switch1/1 -> [STDE_DRV_ENGY_MODE_STATE], Chart/3(E_model)
  Multiport Switch/1 -> Chart/4(D_model), [STDE_DRV_DYN_MODE_STATE]
  油门信号/1 -> Chart/1(throttle)
  制动信号/1 -> Chart/2(brake)
  Chart/1(Model) -> Scope/1, Model/1
  [SOC] -> Chart/5(SOC)
  HEV1/1 -> Multiport Switch1/3
  EV1/1 -> Multiport Switch1/2
  [E_model] -> Multiport Switch1/1

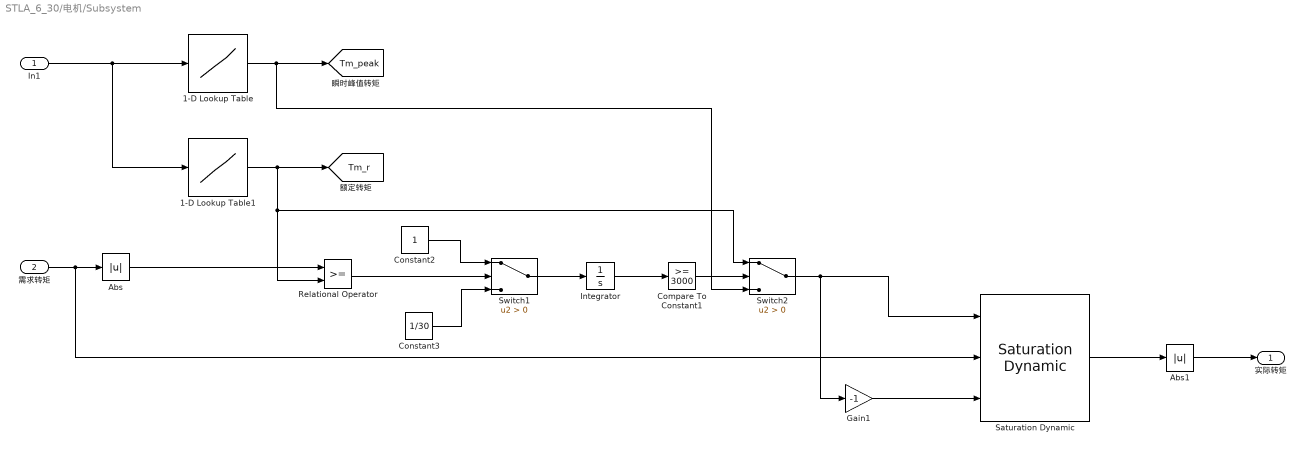
== system STLA_6_30/电机/Subsystem ==
  In1 : Inport
  需求转矩 : Inport  Port=2
  1-D Lookup Table : Lookup_n-D  NumberOfTableDimensions=1  BreakpointsForDimension1="[ 0   1000  2000  3030  4000  5000  6000  8000  10000  12000  14000]"  Table="[110  110   110   110   83.6  66.9  55.7  41.8  33.4   27.9   23.9]"  InternalRulePriority=Speed  RndMeth=Simplest
  1-D Lookup Table1 : Lookup_n-D  NumberOfTableDimensions=1  BreakpointsForDimension1="[ 0   1000  2000  3030  4000  5000  6000  8000  10000  12000  14000]"  Table="[30   30    30    30    30    30    30    30    30     30     27.9]"  InternalRulePriority=Speed  RndMeth=Simplest
  Abs : Abs  SaturateOnIntegerOverflow=off
  Abs1 : Abs  SaturateOnIntegerOverflow=off
  Compare To Constant1 : simulink/Logic and Bit Operations/Compare To Constant  relop=>=  const=3000  OutDataTypeStr=boolean  ZeroCross=off
  Constant2 : Constant
  Constant3 : Constant  Value=1/30
  Gain1 : Gain  Gain=-1
  Integrator : Integrator  LimitOutput=on  UpperSaturationLimit=10  LowerSaturationLimit=0  ZeroCross=off
  Relational Operator : RelationalOperator  OutDataTypeStr=boolean  ZeroCross=off  RndMeth=Simplest  InputSameDT=off
  Saturation Dynamic : simulink/Discontinuities/Saturation Dynamic  OutMin=[]  OutMax=[]  OutDataTypeStr=Inherit: Same as second input  OutDataType=fixdt(1, 16)  OutScaling=2^-10  DoSatur=off
  Switch1 : Switch  Criteria=u2 > Threshold  SaturateOnIntegerOverflow=off  InputSameDT=off
  Switch2 : Switch  Criteria=u2 > Threshold  SaturateOnIntegerOverflow=off  InputSameDT=off
  实际转矩 : Outport
  tag scope: Tm_peak=global, Tm_r=global
  wires:
  需求转矩/1 -> Saturation Dynamic/2, Abs/1
  Switch2/1 -> Saturation Dynamic/1, Gain1/1
  Gain1/1 -> Saturation Dynamic/3
  1-D Lookup Table/1 -> Switch2/3, [Tm_peak]
  In1/1 -> 1-D Lookup Table1/1, 1-D Lookup Table/1
  Relational Operator/1 -> Switch1/2
  1-D Lookup Table1/1 -> Switch2/1, Relational Operator/2, [Tm_r]
  Switch1/1 -> Integrator/1
  Abs/1 -> Relational Operator/1
  Compare To Constant1/1 -> Switch2/2
  Constant3/1 -> Switch1/3
  Constant2/1 -> Switch1/1
  Integrator/1 -> Compare To Constant1/1
  Saturation Dynamic/1 -> Abs1/1
  Abs1/1 -> 实际转矩/1

== system STLA_6_30/电池/Subsystem ==
  电流 : Inport
  " " : Gain  Gain=10
  Constant : Constant  Value=10
  Constant1 : Constant  Value=25
  Gain1 : Gain  Gain=1/117000
  Integrator : Integrator  InitialCondition=25
  Saturation : Saturate  UpperLimit=190  LowerLimit=-40
  Square : Math  Operator=square
  Sum : Sum  Inputs=|+-
  Sum1 : Sum  Inputs=|+-
  总内阻 : Gain  Gain=0.54
  温度 : Outport
  wires:
  Square/1 -> 总内阻/1
  Sum/1 -> " "/1
  总内阻/1 -> Sum1/1
  " "/1 -> Sum1/2
  Sum1/1 -> Gain1/1
  Gain1/1 -> Integrator/1
  Integrator/1 -> Saturation/1
  Saturation/1 -> Sum/1, 温度/1
  Constant1/1 -> Sum/2
  电流/1 -> Square/1

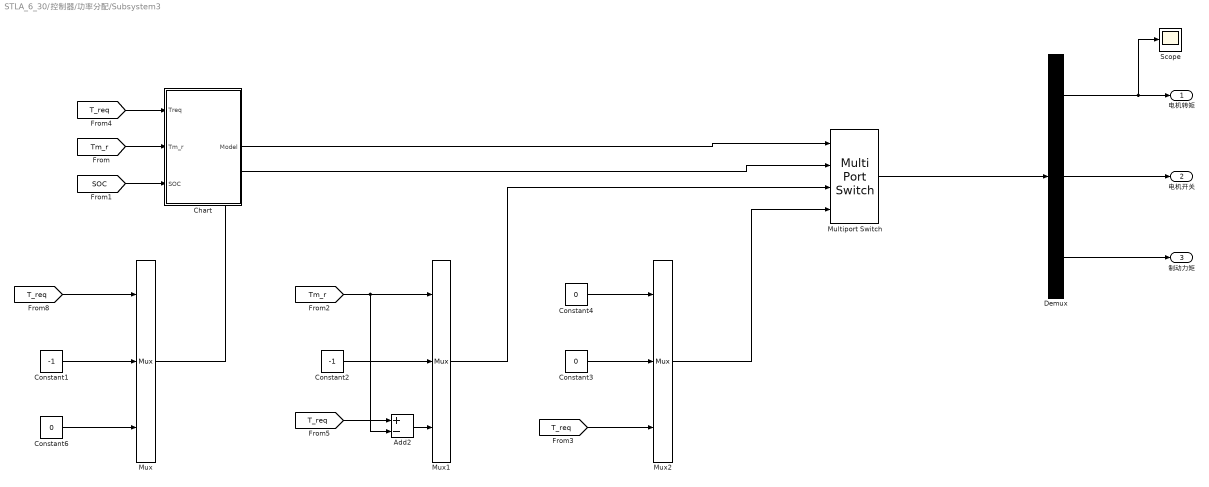
== system STLA_6_30/控制器/功率分配/Subsystem3 ==
  Add2 : Sum  Inputs=+-
  Chart : Stateflow chart  TreatAsAtomicUnit=on
  Constant1 : Constant  Value=-1
  Constant2 : Constant  Value=-1
  Constant3 : Constant  Value=0
  Constant4 : Constant  Value=0
  Constant6 : Constant  Value=0
  Demux : Demux  Outputs=3
  Multiport Switch : MultiPortSwitch  SaturateOnIntegerOverflow=off  InputSameDT=off
  Mux : Mux  Inputs=3
  Mux1 : Mux  Inputs=3
  Mux2 : Mux  Inputs=3
  Scope : Scope
      settings: ActiveDisplayYMinimum=-1  ActiveDisplayYMaximum=1  DataLoggingVariableName=ScopeData17  DataLoggingSaveFormat=Array
  电机转矩 : Outport
  电机开关 : Outport  Port=2
  "制动力矩 " : Outport  Port=3
  wires:
  Multiport Switch/1 -> Demux/1
  Mux/1 -> Multiport Switch/2
  Chart/1(Model) -> Multiport Switch/1
  Demux/3 -> "制动力矩 "/1
  Demux/2 -> 电机开关/1
  Demux/1 -> Scope/1, 电机转矩/1
  [T_req] -> Chart/1(Treq)
  [Tm_r] -> Chart/2(Tm_r)
  [SOC] -> Chart/3(SOC)
  [T_req] -> Mux/1
  Constant1/1 -> Mux/2
  Constant6/1 -> Mux/3
  [Tm_r] -> Mux1/1, Add2/2
  Constant2/1 -> Mux1/2
  Add2/1 -> Mux1/3
  [T_req] -> Add2/1
  [T_req] -> Mux2/3
  Constant3/1 -> Mux2/2
  Constant4/1 -> Mux2/1
  Mux1/1 -> Multiport Switch/3
  Mux2/1 -> Multiport Switch/4

== stateflow chart STLA_6_30/控制器/功率分配/Subsystem3/Chart ==
  state model1
    entry:
    Model=1;
  state model2
    entry:
    Model=2;
  state model3
    entry:
    Model=3;
  (default) -> model1
  model1 -> (junction 4) : [(Treq<Tm_r&SOC<0.9)==0]
  (junction 4) -> model1 [order 1] : [Treq<Tm_r&SOC<0.9]
  (junction 4) -> model2 [order 2] : [Treq>=Tm_r&SOC<0.9]
  model2 -> (junction 4) : [(Treq>=Tm_r&SOC<0.9)==0]
  (junction 4) -> model3 [order 3] : [SOC>=0.9]
  model3 -> (junction 4) : [(SOC>=0.9)==0]
  data: Treq input; Model output; Tm_r input; SOC input

== stateflow chart STLA_6_30/控制器/模式选择/Chart ==
  state Brake1
    entry:
    Model=2;
  state EV_ECO
    entry:
    Model=3;
  state stop
    entry:
    Model=1;
  state HEV_Charge
    entry:
    Model=9;
  state EV_Comfort
    entry:
    Model=4;
  state HEV_Sport
    entry:
    Model=8;
  state EV_Sport
    entry:
    Model=5;
  state HEV_Comfort
    entry:
    Model=7;
  state HEV_ECO
    entry:
    Model=6;
  (default) -> stop
  stop -> (junction 3) : [throttle>1e-4|brake>1e-4]
  (junction 3) -> stop [order 2] : [throttle<1e-4&brake<1e-4]
  (junction 3) -> Brake1 [order 3] : [throttle<1e-4&brake>1e-4]
  Brake1 -> (junction 3) : [(throttle<1e-4&brake>1e-4)==0]
  EV_ECO -> (junction 3) : [(throttle>1e-4&brake<1e-4&E_model==0&D_model==0&SOC>0.2)==0]
  (junction 3) -> EV_ECO [order 4] : [throttle>1e-4&brake<1e-4&E_model==0&D_model==0&SOC>0.2]
  (junction 3) -> HEV_Charge [order 9] : [throttle>1e-4&brake<1e-4&SOC<=0.2]
  HEV_Charge -> (junction 3) : [(throttle>1e-4&brake<1e-4&SOC<=0.2)==0]
  (junction 3) -> EV_Comfort [order 5] : [throttle>1e-4&brake<1e-4&E_model==0&D_model==1&SOC>0.2]
  EV_Sport -> (junction 3) : [(throttle>1e-4&brake<1e-4&E_model==0&D_model==2&SOC>0.2)==0]
  (junction 3) -> HEV_Sport [order 1] : [throttle>1e-4&brake<1e-4&E_model==1&D_model==2&SOC>0.2]
  EV_Comfort -> (junction 3) : [(throttle>1e-4&brake<1e-4&E_model==0&D_model==1&SOC>0.2)==0]
  (junction 3) -> EV_Sport [order 6] : [throttle>1e-4&brake<1e-4&E_model==0&D_model==2&SOC>0.2]
  HEV_ECO -> (junction 3) : [(throttle>1e-4&brake<1e-4&E_model==1&D_model==0&SOC>0.2)==0]
  HEV_Sport -> (junction 3) : [(throttle>1e-4&brake<1e-4&E_model==1&D_model==2&SOC>0.2)==0]
  (junction 3) -> HEV_Comfort [order 8] : [throttle>1e-4&brake<1e-4&E_model==1&D_model==1&SOC>0.2]
  HEV_Comfort -> (junction 3) : [(throttle>1e-4&brake<1e-4&E_model==1&D_model==1&SOC>0.2)==0]
  (junction 3) -> HEV_ECO [order 7] : [throttle>1e-4&brake<1e-4&E_model==1&D_model==0&SOC>0.2]
  data: throttle input; brake input; Model output; E_model input; D_model input; SOC input

== stateflow chart STLA_6_30/控制器/挡位切换/Chart ==
  state D
    state D1
      entry:
      ratio=3.8;
      gear=2;
    state D2
      entry:
      ratio=2.2;
      gear=3;
    state D3
      entry:
      ratio=1.4;
      gear=4;
    state D4
      entry:
      ratio=1;
      gear=5;
    state D5
      entry:
      ratio=0.8;
      gear=6;
    state D6
      entry:
      ratio=0.7;
      gear=7;
    state D7
      entry:
      ratio=0.6;
      gear=8;
    (default) -> D1
    D2 -> D3 [order 1] : [V>=50]
    D3 -> D4 [order 2] : [V>=70]
    D4 -> D5 [order 2] : [V>=90]
    D5 -> D6 [order 2] : [V>=120]
    D1 -> D2 : [V>=25]
    D6 -> D7 [order 2] : [V>=150]
    D5 -> D4 [order 1] : [V<=85]
    D7 -> D6 : [V<=135]
    D4 -> D3 [order 1] : [V<=65]
    D3 -> D2 [order 1] : [V<=45]
    D6 -> D5 [order 1] : [V<=115]
    D2 -> D1 [order 2] : [V<=20]
  state P_N
    state P
      entry:
      gear=0;
    state N
      entry:
      gear=1;
    (default) -> P
    P -> N : [PN_flag==0]
    N -> P : [PN_flag==1]
  (default) -> P_N
  P_N -> D : [throttle>1e-4|brake>1e-4]
  D -> P_N : [throttle<1e-4&brake<1e-4&T_ct>=20]
  data: brake input; throttle input; gear output; ratio output; V input; PN_flag input; T_ct input
